simulink model "OldSimulink_SerialBlockExample"  (R2025b)
settings: Solver=FixedStepAuto  StartTime=0.0  StopTime=inf  FixedStep=0.001  RelTol=1e-3
undefined symbols (not defined in the file): LF
libraries: instrumentseriallib x4, simulink x2
settings Model: Creator=talles  LastModifiedBy=ajax

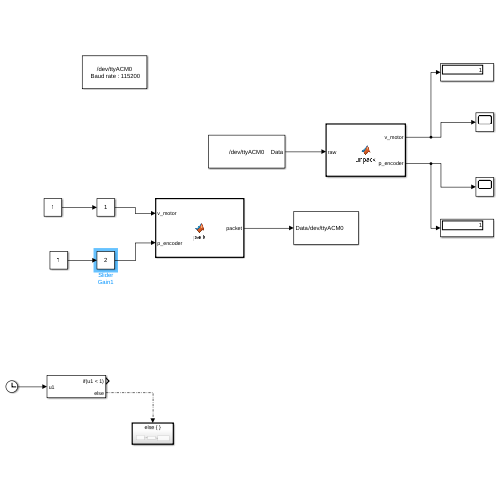
[thumbnail: Simulink's stored preview of the top-level diagram]
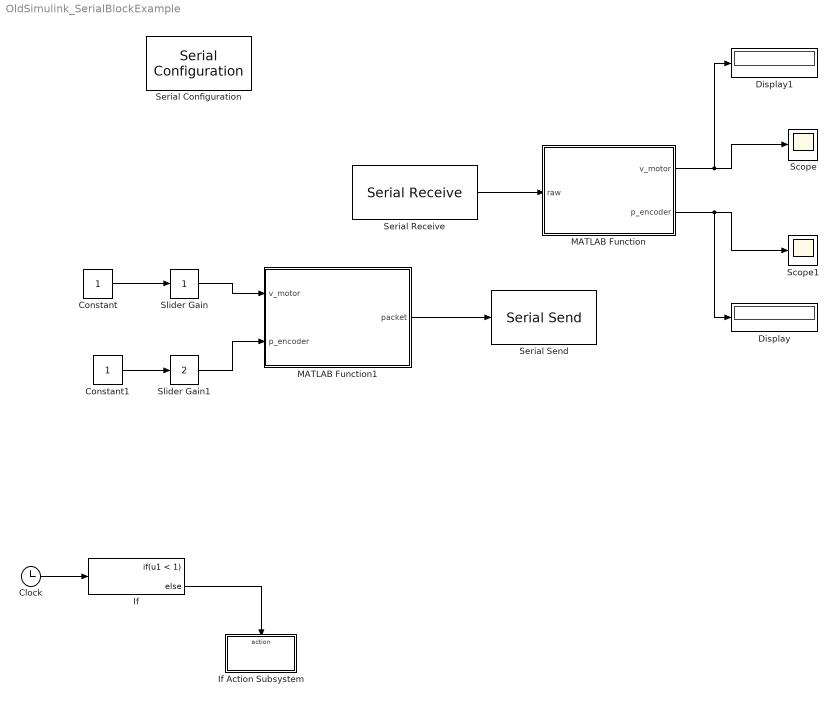
== system OldSimulink_SerialBlockExample ==
  Clock : Clock
  Constant : Constant
  Constant1 : Constant
  Display : Display
  Display1 : Display
  If : If  IfExpression=u1 < 1
  If Action Subsystem : Subsystem  TreatAsAtomicUnit=on
  MATLAB Function : MATLAB Function  TreatAsAtomicUnit=on
  MATLAB Function1 : MATLAB Function  TreatAsAtomicUnit=on
  Scope : Scope
  Scope1 : Scope
      settings: ActiveDisplayYMinimum=0.9  ActiveDisplayYMaximum=1.1
  Serial Configuration : instrumentseriallib/Serial Configuration  Priority=-200000  PortSel=/dev/ttyACM0  Port=/dev/ttyACM0  ComPort=/dev/ttyACM0  BaudRate=115200  DataBits=8  Parity=none  StopBits=1  ByteOrder=little-endian  FlowControl=none  Timeout=0.0001  SimulateUsing=Interpreted execution  BlockInModel=on  aMode=1
      settings: LibrarySourceBlock=embeddedtargetslib/Host Communication/Serial Configuration
  Serial Receive : instrumentseriallib/Serial Receive  Priority=1  PortSel=/dev/ttyACM0  Port=/dev/ttyACM0  ComPort=/dev/ttyACM0  DataType=uint8  SaveDataType=uint8  ToggleHeader=on  Header=['#']  ToggleDataSize=on  DataSize=[1 18]  ToggleTerminator=on  Terminator=LF ('\n')  CustomTerminator=[]  InputFormat=Column major  EnableBlockingMode=on  ActionDataUnavailable=Output last received value  ActionWhenDataUnavailable=Output last received value  CustomValue=0  SampleTime=0.01  SimulateUsing=Interpreted execution  BlockInModel=on  aMode=1  LibraryInUse=instrumentlib
  Serial Send : instrumentseriallib/Serial Send  Priority=1  PortSel=/dev/ttyACM0  Port=/dev/ttyACM0  ComPort=/dev/ttyACM0  Header=['#']  Terminator=LF ('\n')  CustomTerminator=[]  EnableBlockingMode=on  SimulateUsing=Interpreted execution  BlockInModel=on  aMode=1
      settings: LibrarySourceBlock=embeddedtargetslib/Host Communication/Serial Send
  Slider Gain : simulink/Math Operations/Slider Gain  gain=1  low=0  high=2
  Slider Gain1 : simulink/Math Operations/Slider Gain  gain=2  low=0  high=2
  wires:
  Clock/1 -> If/1
  If/2 -> If Action Subsystem/Action
  MATLAB Function1/1(packet) -> Serial Send/1
  Slider Gain/1 -> MATLAB Function1/1(v_motor)
  Slider Gain1/1 -> MATLAB Function1/2(p_encoder)
  Constant1/1 -> Slider Gain1/1
  Constant/1 -> Slider Gain/1
  MATLAB Function/2(p_encoder) -> Display/1, Scope1/1
  MATLAB Function/1(v_motor) -> Display1/1, Scope/1
  Serial Receive/1 -> MATLAB Function/1(raw)

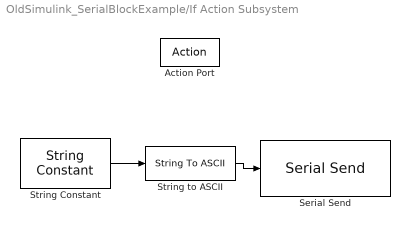
== system OldSimulink_SerialBlockExample/If Action Subsystem ==
  Action Port : ActionPort  ActionPortLabel=else
  Serial Send : instrumentseriallib/Serial Send  Priority=1  PortSel=/dev/ttyACM0  Port=/dev/ttyACM0  ComPort=/dev/ttyACM0  Header=[]  Terminator=LF ('\n')  CustomTerminator=[]  EnableBlockingMode=on  SimulateUsing=Interpreted execution  BlockInModel=on  aMode=1
  String Constant : StringConstant  String="\"1111,5556\""
  String to ASCII : StringToASCII
  wires:
  String Constant/1 -> String to ASCII/1
  String to ASCII/1 -> Serial Send/1

== matlab function OldSimulink_SerialBlockExample/MATLAB Function ==
  data: raw input; v_motor output; p_encoder output
function [v_motor, p_encoder] = unpack(raw)

% Cast inputs and outputs explicitly so Simulink can infer types
str = char(raw(:)');

vals = sscanf(str(2:end), '%d,%d');

% Force scalar double outputs — Simulink needs this to be unambiguous
if numel(vals) >= 2
    v_motor   = double(vals(1));
    p_encoder = double(vals(2));
else
    v_motor   = double(0);
    p_encoder = double(0);
end

== matlab function OldSimulink_SerialBlockExample/MATLAB Function1 ==
  data: v_motor input; packet output; p_encoder input
function packet = pack(v_motor, p_encoder)

str = sprintf('#%+07d,%+07d\n', int32(v_motor), int32(p_encoder));

% Tell Simulink: packet is always exactly 18 uint8 elements
packet = uint8(zeros(1, 17));
for i = 1:17
    packet(i) = uint8(str(i));
end
